simulink model "Test"  (R2022a)
settings: Solver=FixedStepAuto  StartTime=0.0  StopTime=500  RelTol=1e-3
undefined symbols (not defined in the file or in its folder): InputPWM, WheelSpeed
libraries: arduinolib x21, mobileRoboticsTrainingLib x2
settings Model: ExtModeTrigDuration=2  Creator=sarah  LastModifiedBy=sarah
settings OptimizationCC: EnhancedBackFolding=on  PassReuseOutputArgsAs=Individual arguments  ZeroExternalMemoryAtStartup=off  ZeroInternalMemoryAtStartup=off  MaxStackSize=64  OptimizeBlockOrder=speed  DifferentSizesBufferReuse=on  OptimizationCustomize=off  EfficientTunableParamExpr=on
settings DebuggingCC: MultiTaskDSMMsg=none  ParameterTunabilityLossMsg=error
settings HardwareCC: ProdBitPerPointer=32  ProdBitPerSizeT=32  ProdBitPerPtrDiffT=32  ProdLargestAtomicInteger=Long  ProdLargestAtomicFloat=Double  ProdWordSize=32  ProdHWDeviceType=ARM Compatible->ARM Cortex  UseEmbeddedCoderFeatures=off  UseSimulinkCoderFeatures=off
settings SFSimCC: MATLABDynamicMemAlloc=off
settings RTWCC: SystemTargetFile=ert.tlc  HardwareBoard=Arduino Nano 33 IoT  TemplateMakefile=ert_default_tmf  Toolchain=Arduino ARM
settings CodeAppCC: ForceParamTrailComments=on  IgnoreCustomStorageClasses=off  OperatorAnnotations=on  SimulinkDataObjDesc=on  SFDataObjDesc=on  InsertBlockDesc=on
settings ERTTargetCC: SupportContinuousTime=on  SupportNonInlinedSFcns=on  SupportVariableSizeSignals=on  ExtModeTransport=3  ExtModeStaticAlloc=on  ExtModeStaticAllocSize=8192  ExtModeMexFile=ext_xcp  ExtModeIntrfLevel=Level2 - Open

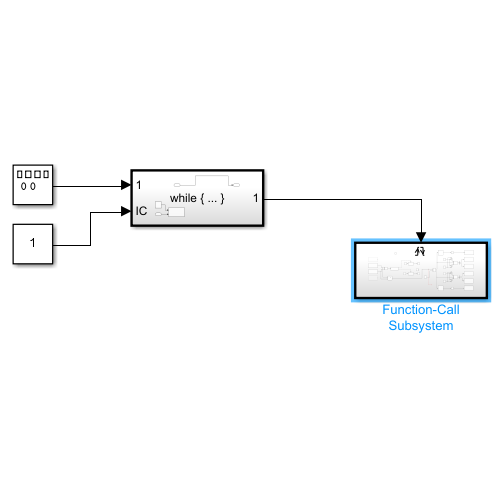
[thumbnail: Simulink's stored preview of the top-level diagram]
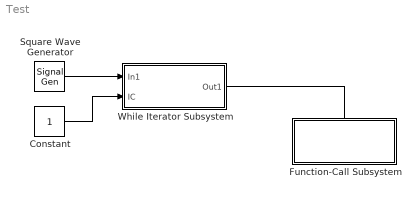
== system Test ==
  Constant : Constant
  Function-Call Subsystem : Subsystem  TreatAsAtomicUnit=on
  Square Wave Generator : SignalGenerator  WaveForm=square  Units=rad/sec
  While Iterator Subsystem : Subsystem  TreatAsAtomicUnit=on
  wires:
  Square Wave Generator/1 -> While Iterator Subsystem/1(In1)
  Constant/1 -> While Iterator Subsystem/2(IC)
  While Iterator Subsystem/1(Out1) -> ?

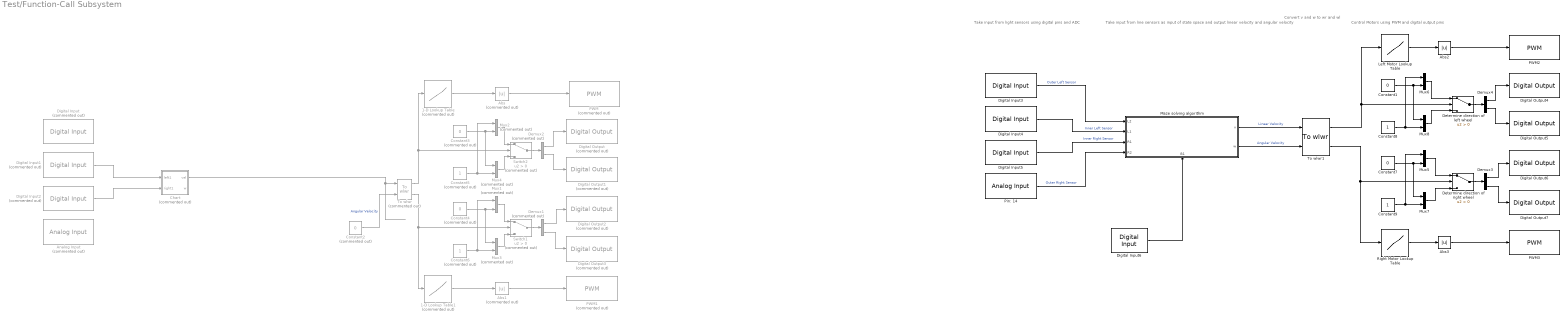
== system Test/Function-Call Subsystem ==
  note: Take input from line sensors as input of state space and output
      | linear velocity and angular velocity
  note: Take input from light sensors using
      | digital pins and ADC
  note: Convert v and w to
      | wr and wl
  note: Control Motors using PWM and digital output pins
  1-D Lookup Table : Lookup_n-D  Commented=on  NumberOfTableDimensions=1  BreakpointsForDimension1=WheelSpeed  Table=InputPWM  InternalRulePriority=Speed  RndMeth=Simplest
  1-D Lookup Table1 : Lookup_n-D  Commented=on  NumberOfTableDimensions=1  BreakpointsForDimension1=WheelSpeed  Table=InputPWM  InternalRulePriority=Speed  RndMeth=Simplest
  Abs : Abs  Commented=on  SaturateOnIntegerOverflow=off
  Abs1 : Abs  Commented=on  SaturateOnIntegerOverflow=off
  Abs2 : Abs  SaturateOnIntegerOverflow=off
  Abs3 : Abs  SaturateOnIntegerOverflow=off
  Analog Input : arduinolib/Analog Input  Commented=on  pinNumber=0  ReadResultsOnly=off  ConversionTriggerSource=Software  ExternalTriggerType=uint32( 0 )  OutputDataType=uint16  EnableConversionCompleteNotify=off  EnableOuputStatus=off  SampleTime=-1  blockPlatform=arduino
  Chart : Stateflow chart  Commented=on  TreatAsAtomicUnit=on
  Constant1 : Constant  Value=0
  Constant2 : Constant  Commented=on  Value=0
  Constant3 : Constant  Commented=on  Value=0
  Constant4 : Constant  Commented=on  Value=0
  Constant5 : Constant  Commented=on
  Constant6 : Constant  Commented=on
  Constant7 : Constant  Value=0
  Constant8 : Constant
  Constant9 : Constant
  Demux1 : Demux  Commented=on  Outputs=2
  Demux2 : Demux  Commented=on  Outputs=2
  Demux3 : Demux  Outputs=2
  Demux4 : Demux  Outputs=2
  Determine direction of left wheel : Switch  Criteria=u2 > Threshold  SaturateOnIntegerOverflow=off  InputSameDT=off
  Determine direction of right wheel : Switch  Criteria=u2 > Threshold  SaturateOnIntegerOverflow=off  InputSameDT=off
  Digital Input : arduinolib/Digital Input  Commented=on  pinNumber=8  mode=Default  Direction=input  SampleTime=0.1  blockPlatform=arduino
  Digital Input1 : arduinolib/Digital Input  Commented=on  pinNumber=11  mode=Default  Direction=input  SampleTime=-1  blockPlatform=arduino
  Digital Input2 : arduinolib/Digital Input  Commented=on  pinNumber=12  mode=Default  Direction=input  SampleTime=-1  blockPlatform=arduino
  Digital Input3 : arduinolib/Digital Input  pinNumber=8  mode=Default  Direction=input  SampleTime=0.1  blockPlatform=arduino
  Digital Input4 : arduinolib/Digital Input  pinNumber=11  mode=Default  Direction=input  SampleTime=-1  blockPlatform=arduino
  Digital Input5 : arduinolib/Digital Input  pinNumber=12  mode=Default  Direction=input  SampleTime=-1  blockPlatform=arduino
  Digital Input6 : arduinolib/Digital Input  pinNumber=13  mode=Default  Direction=input  SampleTime=0.1  blockPlatform=arduino
  Digital Output : arduinolib/Digital Output  Commented=on  pinNumber=6  Direction=output  blockPlatform=arduino
  Digital Output1 : arduinolib/Digital Output  Commented=on  pinNumber=7  Direction=output  blockPlatform=arduino
  Digital Output2 : arduinolib/Digital Output  Commented=on  pinNumber=4  Direction=output  blockPlatform=arduino
  Digital Output3 : arduinolib/Digital Output  Commented=on  pinNumber=5  Direction=output  blockPlatform=arduino
  Digital Output4 : arduinolib/Digital Output  pinNumber=6  Direction=output  blockPlatform=arduino
  Digital Output5 : arduinolib/Digital Output  pinNumber=7  Direction=output  blockPlatform=arduino
  Digital Output6 : arduinolib/Digital Output  pinNumber=4  Direction=output  blockPlatform=arduino
  Digital Output7 : arduinolib/Digital Output  pinNumber=5  Direction=output  blockPlatform=arduino
  Left Motor Lookup Table : Lookup_n-D  NumberOfTableDimensions=1  BreakpointsForDimension1=WheelSpeed  Table=InputPWM  InternalRulePriority=Speed  RndMeth=Simplest
  Maze solving algorithm : Stateflow chart  TreatAsAtomicUnit=on
      settings: PortSchema="{\"entries\":[{\"content\":{\"sides\":[{\"content\":{\"connectorIds\":[\"In2\",\"In3\",\"In5\",\"In4\"]},\"type\":\"ConnectorPlacement.EquallySpacedRectSide\",\"uuid\":\"aba539e4-9d8a-47f4-8547-39721ab9b9f4\"},{\"content\":{\"connectorIds\":[\"Out1\",\"Out2\"],\"side\":\"RIGHT\"},\"type\":\"ConnectorPlacement.EquallySpacedRectSide\",\"uuid\":\"a712b855-a14f-4e8e-9130-f7ec9592e6f1\"},{\"content\":{\"connectorIds\":[],\"side\":\"TOP\"},\"type\":\"ConnectorPlacement.EquallySpacedRectSide\",\"uuid\":\"45676f86-2ce0-4f9f-a8d0-692eeac24e11\"},{\"content\":{\"connectorIds\":[\"In1\"],\"side\":\"BOTTOM\"},\"type\":\"ConnectorPlacement.EquallySpacedRectSide\",\"uuid\":\"12a16515-1ae9-4ad8-8460-42ed0e0f58e0\"}]},\"type\":\"ConnectorPlacement.EquallySpacedConnector\",\"uuid\":\"1c93e922-51ef-4d8f-b0c3-81b6bdc53155\"}],\"packageUris\":[\"http://schema.mathworks.com/mf0/Connector/R2020b\"],\"version\":\"1.0\"}"
  Mux{1..4} (4 alike) : Mux  Commented=on  Inputs=2
  Mux{5..8} (4 alike) : Mux  Inputs=2
  PWM : arduinolib/PWM  Commented=on  pinNumber=2  frequencyType=Default  desiredFrequency=490.2  achievableFrequency=490.2
  PWM1 : arduinolib/PWM  Commented=on  pinNumber=3  frequencyType=Default  desiredFrequency=490.2  achievableFrequency=490.2
  PWM2 : arduinolib/PWM  pinNumber=2  frequencyType=Default  desiredFrequency=490.2  achievableFrequency=490.2
  PWM3 : arduinolib/PWM  pinNumber=3  frequencyType=Default  desiredFrequency=490.2  achievableFrequency=490.2
  Pin: 14 : arduinolib/Analog Input  pinNumber=0  ReadResultsOnly=off  ConversionTriggerSource=Software  ExternalTriggerType=uint32( 0 )  OutputDataType=uint16  EnableConversionCompleteNotify=off  EnableOuputStatus=off  SampleTime=-1  blockPlatform=arduino
  "Right Motor Lookup Table " : Lookup_n-D  NumberOfTableDimensions=1  BreakpointsForDimension1=WheelSpeed  Table=InputPWM  InternalRulePriority=Speed  RndMeth=Simplest
  Switch1 : Switch  Commented=on  Criteria=u2 > Threshold  SaturateOnIntegerOverflow=off  InputSameDT=off
  Switch2 : Switch  Commented=on  Criteria=u2 > Threshold  SaturateOnIntegerOverflow=off  InputSameDT=off
  To wlwr : mobileRoboticsTrainingLib/To wlwr  Commented=on  axleLength=axleLength  wheelR=wheelR
  To wlwr1 : mobileRoboticsTrainingLib/To wlwr  axleLength=axleLength  wheelR=wheelR
  wires:
  Digital Input1/1 -> Chart/1(left1)
  Digital Input2/1 -> Chart/2(right1)
  1-D Lookup Table/1 -> Abs/1
  1-D Lookup Table1/1 -> Abs1/1
  Switch2/1 -> Demux2/1
  Demux2/2 -> Digital Output1/1
  Abs/1 -> PWM/1
  Mux2/1 -> Switch2/1
  To wlwr/1 -> 1-D Lookup Table/1, Switch2/2
  Demux1/1 -> Digital Output2/1
  Mux4/1 -> Switch2/3
  Constant4/1 -> Mux3/1, Mux1/2
  Mux1/1 -> Switch1/1
  Constant6/1 -> Mux1/1, Mux3/2
  To wlwr/2 -> Switch1/2, 1-D Lookup Table1/1
  Constant2/1 -> To wlwr/2  "Angular Velocity"
  Demux1/2 -> Digital Output3/1
  Abs1/1 -> PWM1/1
  Demux2/1 -> Digital Output/1
  Switch1/1 -> Demux1/1
  Mux3/1 -> Switch1/3
  Constant3/1 -> Mux4/1, Mux2/2
  Constant5/1 -> Mux2/1, Mux4/2
  Chart/1(vel) -> To wlwr/1
  Mux6/1 -> Determine direction of left wheel/1
  Pin: 14/1 -> Maze solving algorithm/4(R2)  "Outer Right Sensor"
  Digital Input4/1 -> Maze solving algorithm/3(L1)  "Inner Left Sensor"
  Mux7/1 -> Determine direction of right wheel/3
  Constant9/1 -> Mux5/1, Mux7/2
  Abs2/1 -> PWM2/1
  Digital Input5/1 -> Maze solving algorithm/5(R1)  "Inner Right Sensor"
  Demux4/1 -> Digital Output4/1
  Demux4/2 -> Digital Output5/1
  Demux3/1 -> Digital Output6/1
  Determine direction of right wheel/1 -> Demux3/1
  Abs3/1 -> PWM3/1
  Constant8/1 -> Mux6/1, Mux8/2
  To wlwr1/1 -> Left Motor Lookup Table/1, Determine direction of left wheel/2
  Demux3/2 -> Digital Output7/1
  Constant1/1 -> Mux8/1, Mux6/2
  "Right Motor Lookup Table "/1 -> Abs3/1
  Determine direction of left wheel/1 -> Demux4/1
  To wlwr1/2 -> Determine direction of right wheel/2, "Right Motor Lookup Table "/1
  Constant7/1 -> Mux7/1, Mux5/2
  Maze solving algorithm/1(v) -> To wlwr1/1  "Linear Velocity"
  Mux8/1 -> Determine direction of left wheel/3
  Left Motor Lookup Table/1 -> Abs2/1
  Mux5/1 -> Determine direction of right wheel/1
  Digital Input3/1 -> Maze solving algorithm/2(L2)  "Outer Left Sensor"
  Maze solving algorithm/2(w) -> To wlwr1/2  "Angular Velocity"
  Digital Input6/1 -> Maze solving algorithm/1(B1)

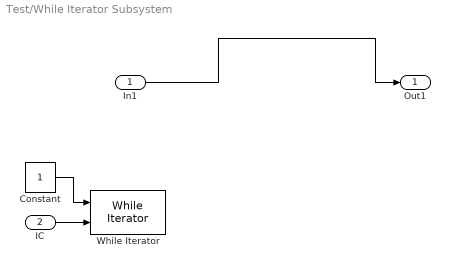
== system Test/While Iterator Subsystem ==
  In1 : Inport
  IC : Inport  Port=2
  Constant : Constant
  While Iterator : WhileIterator
  Out1 : Outport
  wires:
  IC/1 -> While Iterator/2
  In1/1 -> Out1/1
  Constant/1 -> While Iterator/1

== stateflow chart Test/Function-Call Subsystem/Maze solving algorithm ==
  state AdjustRight
    entry:
    v = 0;
    w = 1.4;
  state TurnAround
    entry:
    v = 0;
    state Turn
      entry:
      w = 1.2;
    state Stop1
      entry:
      w = 0;
      done = 1;
    (default) -> TurnAround.Turn
    TurnAround.Turn -> Stop1 : [R1 == 0]
  state AdjustLeft
    entry:
    v = 0;
    w = -1.4;
  state Wait
    entry:
    v = 0;
    w = 0;
  state DeadReckoning
    entry:
    v = 0.1;
    w = 0.05;
  state Start
    entry:
    v = 0.1;
    w = 0.06;
    done = 0;
  state TurnRight1
    entry:
    done = 0;
    state Turn
      entry:
      w = 1.2;
    state Check
      entry:
      w = 1.2;
      check = 1;
      exit:
      check = 0;
    state TurnAgain
      entry:
      w = 1.2;
    state Stop
      entry:
      w = 0;
      done = 1;
    (default) -> TurnRight1.Turn
    TurnRight1.Turn -> Check : [after(0.3,sec)]
    Check -> TurnAgain : [after(0.5,sec)]
    TurnAgain -> TurnRight1.Stop : [R1 == 0]
  state TurnLeft
    entry:
    done = 0;
    state Turn
      entry:
      w = -1.2;
    state Stop
      entry:
      w = 0;
      done = 1;
    (default) -> TurnLeft.Turn
    TurnLeft.Turn -> TurnLeft.Stop : [~R1||~L1]
  state Forward
    state Move
      entry:
      v = 0.1;
      w = 0;
    state Stop
      entry:
      v = 0;
      w = 0;
      done = 1;
    (default) -> Forward.Move
    Forward.Move -> Forward.Stop : [after(0.1,sec)]
  state ForwardMore
    entry:
    done = 0;
    state Move
      entry:
      v = 0.12;
      w = 0.06;
    state Stop
      entry:
      v = 0;
      w = 0;
      done = 1;
    (default) -> ForwardMore.Move
    ForwardMore.Move -> ForwardMore.Stop : [after(0.8,sec)]
  state Stop
    entry:
    v = 0;
    w = 0;
  DeadReckoning -> AdjustRight [order 3] : [R2 == 0]
  AdjustRight -> (junction 295) [order 2] : [after(0.5,sec)]
  AdjustLeft -> (junction 295) [order 2] : [after(0.5,sec)]
  (junction 295) -> TurnAround : [L2&&L1&&R1&&R2]
  DeadReckoning -> AdjustLeft [order 2] : [L2 == 0]
  (default) -> Wait : %start
  Start -> AdjustLeft [order 1] : [L2&&~L1&&R1&&R2]
  AdjustLeft -> Start [order 1] : [(L1&&R1)==0]
  Start -> AdjustRight [order 2] : [L2&&L1&&~R1&&R2]
  AdjustRight -> Start [order 1] : [(L1&&R1)==0]
  Start -> TurnAround [order 4] : [L2&&L1&&R1&&R2]
  TurnAround -> Start : [done == 1]
  Wait -> Start : [B1 == 1]
  DeadReckoning -> Start [order 1] : [(L1&&R1)==0]
  TurnRight1 -> Start [order 1] : [done == 1]
  Start -> Forward [order 3] : [(~L2||~R2)&&~L1&&~R1]
  TurnLeft -> Start : [done == 1]
  ForwardMore -> DeadReckoning [order 2] : [L1&&R1&&done]
  Forward -> TurnRight1 [order 3] : [L2&&~R2&&done]
  Forward -> TurnLeft [order 2] : [~L2&&R2&&done]
  ForwardMore -> TurnRight1 [order 3] : [L2&&R2&&(L1||R1)&&done]
  Forward -> ForwardMore [order 1] : [((L2&&R2)||(~L2&&~R2))&&done]
  TurnRight1 -> Stop [order 2] : [~L2&&~L1&&~R1&&~R2&&check]
  ForwardMore -> Stop [order 1] : [~L2&&~L1&&~R1&&~R2&&done]
  data: B1 input; L2 input; L1 input; R2 input; R1 input; v output; w output; done local =0; check local =0

== stateflow chart Test/Function-Call Subsystem/Chart ==
  state Move
    entry:
    vel = 0;
    w = 0;
  state AdjustLeft
    entry:
    vel = 0.1;
    deg = 5;
  state Start
    entry:
    vel = 0.1;
  state AdjustRight1
    entry:
    vel = 0.1;
    deg = -5;
  (default) -> Move : %start
  Move -> Start : [(left1&&right1)==0]
  Start -> AdjustLeft [order 1] : [left2&&~left1&&right1&&right2]
  AdjustLeft -> Start : [(left1&&right1)==0]
  Start -> AdjustRight1 [order 2] : [[left2&&left1&&~right1&&right2]]
  AdjustRight1 -> Start : [(left1&&right1)==0]
  data: left1 input; right1 input; vel output; w output
